simulink subsystem "ABC_to_alpha_beta"  (R2022b)
settings: Solver=VariableStepAuto  StartTime=0.0  StopTime=10.0  RelTol=1e-3
settings Model: Creator=MAAM  LastModifiedBy=MAAM

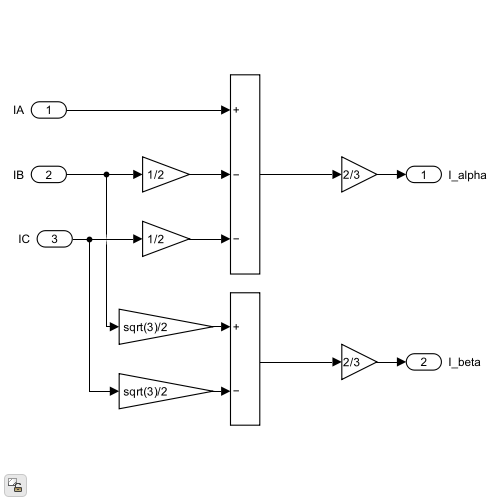
[thumbnail: Simulink's stored preview of the top-level diagram]
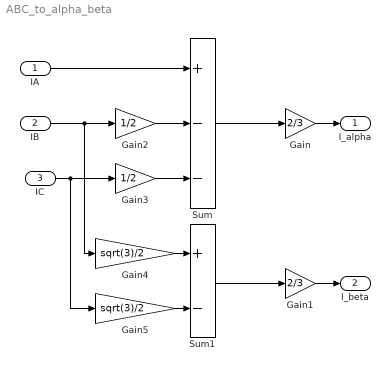
== system ABC_to_alpha_beta ==
  IA : Inport
  IB : Inport  Port=2
  IC : Inport  Port=3
  Gain : Gain  Gain=2/3
  Gain1 : Gain  Gain=2/3
  Gain2 : Gain  Gain=1/2
  Gain3 : Gain  Gain=1/2
  Gain4 : Gain  Gain=sqrt(3)/2
  Gain5 : Gain  Gain=sqrt(3)/2
  Sum : Sum  Inputs=+--
  Sum1 : Sum  Inputs=+-
  I_alpha : Outport
  I_beta : Outport  Port=2
  wires:
  IA/1 -> Sum/1
  Sum1/1 -> Gain1/1
  Sum/1 -> Gain/1
  Gain2/1 -> Sum/2
  IB/1 -> Gain2/1, Gain4/1
  Gain3/1 -> Sum/3
  IC/1 -> Gain3/1, Gain5/1
  Gain4/1 -> Sum1/1
  Gain5/1 -> Sum1/2
  Gain/1 -> I_alpha/1
  Gain1/1 -> I_beta/1
